simulink model "SF043A_TqOscn"  (R2013b)
settings: Solver=FixedStepDiscrete  SolverMode=SingleTasking  StartTime=0.0  StopTime=1  FixedStep=0.002  RelTol=1e-3
values from neighbouring files (symbols this model uses):
  ARCHGLBPRM_2MILLISEC_SEC_F32 = DataDict.Constant    [SF043A_TqOscn_DataDict.m]
  ARCHGLBPRM_2PI_ULS_F32 = DataDict.Constant    [SF043A_TqOscn_DataDict.m]
  DCTHD_MOTNWTMTR_F32 = DataDict.Constant    [SF043A_TqOscn_DataDict.m]
  DFTFALLRAMPRATE_MOTNWTMTRPERSEC_F32 = DataDict.Constant    [SF043A_TqOscn_DataDict.m]
  DFTPHAAGINC_MATRAD_F32 = DataDict.Constant    [SF043A_TqOscn_DataDict.m]
  DFTRISNGRAMPRATE_MOTNWTMTRPERSEC_F32 = DataDict.Constant    [SF043A_TqOscn_DataDict.m]
  FltInj_f32 = DataDict.Client    [SF043A_TqOscn_DataDict.m]
  FLTINJ_TQOSCN_PREFINALCMD = DataDict.Constant    [SF043A_TqOscn_DataDict.m]
  MAXAMP_MOTNWTMTR_F32 = DataDict.Constant    [SF043A_TqOscn_DataDict.m]
  MAXRAMPRATE_MOTNWTMTR_F32 = DataDict.Constant    [SF043A_TqOscn_DataDict.m]
  MINAMP_MOTNWTMTR_F32 = DataDict.Constant    [SF043A_TqOscn_DataDict.m]
  MINRAMPRATE_MOTNWTMTR_F32 = DataDict.Constant    [SF043A_TqOscn_DataDict.m]
  TqOscnAmpLimY = DataDict.Calibration    [SF043A_TqOscn_DataDict.m]
  TqOscnFallRampRateCal = DataDict.Calibration    [SF043A_TqOscn_DataDict.m]
  TqOscnFrqIn = DataDict.Calibration    [SF043A_TqOscn_DataDict.m]
  TqOscnRisngRampRateCal = DataDict.Calibration    [SF043A_TqOscn_DataDict.m]
  TqOscnUseRampRateCal = DataDict.Calibration    [SF043A_TqOscn_DataDict.m]
libraries: NxtrLim x6, simulink x3, NxtrAbslt x3, Fil x2, FixdToFloat x2, autosarlib x1, NxtrMath x1, FloatToFixd x1
(part 1 of 2)
settings Model: PauseTimes=0.5  Creator=hz69by  LastModifiedBy=HZ69BY
settings SolverCC: AutoInsertRateTranBlk=on  InsertRTBMode=Always
settings DataIOCC: LimitDataPoints=off  SaveFormat=Structure  ReturnWorkspaceOutputs=on
settings OptimizationCC: BlockReduction=off  InlineParams=on  ZeroExternalMemoryAtStartup=off  ZeroInternalMemoryAtStartup=off  OptimizeModelRefInitCode=on  LifeSpan=1
settings DebuggingCC: SignalInfNanChecking=error  SignalRangeChecking=warning  UnderspecifiedInitializationDetection=Simplified  SolverPrmCheckMsg=error  InheritedTsInSrcMsg=error  DiscreteInheritContinuousMsg=error  SingleTaskRateTransMsg=error  TasksWithSamePriorityMsg=error  SigSpecEnsureSampleTimeMsg=error  CheckMatrixSingularityMsg=error  ParameterUnderflowMsg=error  ParameterPrecisionLossMsg=error  ParameterTunabilityLossMsg=error  FixptConstUnderflowMsg=warning  FixptConstOverflowMsg=warning  VectorMatrixConversionMsg=error  SignalLabelMismatchMsg=error  UnconnectedInputMsg=error  UnconnectedOutputMsg=error  UnconnectedLineMsg=error  SFcnCompatibilityMsg=error  UniqueDataStoreMsg=warning  BusObjectLabelMismatch=error  RootOutportRequireBusObject=error  AssertControl=DisableAll  ModelReferenceIOMsg=error  ModelReferenceVersionMismatchMessage=warning  ModelReferenceIOMismatchMessage=error  ModelReferenceCSMismatchMessage=warning  ModelReferenceDataLoggingMessage=error  StateNameClashWarn=warning  StrictBusMsg=ErrorOnBusTreatedAsVector  NonBusSignalsTreatedAsBus=error  SFUnexpectedBacktrackingDiag=error  SFInvalidInputDataAccessInChartInitDiag=error  SFNoUnconditionalDefaultTransitionDiag=error  SFTransitionOutsideNaturalParentDiag=error  SFUnconditionalTransitionShadowingDiag=error  SFUndirectedBroadcastEventsDiag=error
settings ModelReferenceCC: ModelReferenceNumInstancesAllowed=Single
settings RTWCC: SystemTargetFile=autosar.tlc  GenCodeOnly=on  TemplateMakefile=ert_default_tmf  Description=AUTOSAR  GenerateReport=on  ProcessScript=autosar_make_rtw_hook  LaunchReport=on
settings CodeAppCC: GenerateComments=off  IgnoreCustomStorageClasses=off  CustomSymbolStrType=$N$R$M  CustomSymbolStrBlkIO=$N$M  SimulinkBlockComments=off
settings STFCustomTargetCC: ParMdlRefBuildCompliant=on  CompOptLevelCompliant=on  IncludeMdlTerminateFcn=off  CombineOutputUpdateFcns=on  SuppressErrorStatus=on  ERTFirstTimeCompliant=on  ERTCustomFileBanners=on  SupportNonFinite=off  SupportComplex=off  SupportContinuousTime=off  SupportNonInlinedSFcns=off  MATLABClassNameForMDSCustomization=Simulink.SoftwareTarget.ERTCustomization  AutosarCompliant=on  GRTInterface=off  SystemTargetFile=autosar.tlc
settings ERTTargetCC: CodeReplacementLibrary=ANSI_C  ConcurrentExecutionCompliant=off  IncludeMdlTerminateFcn=off  SuppressErrorStatus=on  SupportNonFinite=off  SupportComplex=off  ModelStepFunctionPrototypeControlCompliant=off  CPPClassGenCompliant=off  AutosarCompliant=on  InlinedParameterPlacement=NonHierarchical  ERTCustomFileTemplate=example_file_process.tlc  EnableUserReplacementTypes=on

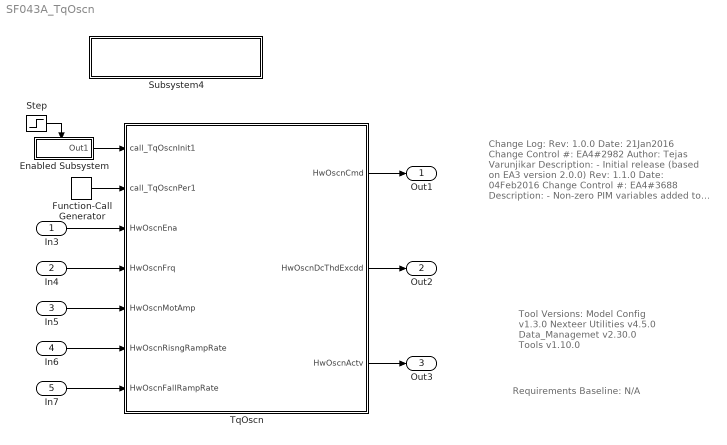
== system SF043A_TqOscn ==
  note: Change Log:
      |
      | Rev: 1.0.0
      | Date: 21Jan2016
      | Change Control #: EA4#2982
      | Author: Tejas Varunjikar
      | Description:
      | - Initial release (based on EA3 version 2.0.0)
      |
      | Rev: 1.1.0
      | Date: 04Feb2016
      | Change Control #: EA4#3688
      | Description:
      | - Non-zero PIM variables added to init
      | - Else logic updated inside "Angle Wrapper" subsystem
  note: Requirements Baseline: N/A
  note: Tool Versions:
      |
      | Model Config v1.3.0
      | Nexteer Utilities v4.5.0
      | Data_Managemet v2.30.0
      | Tools v1.10.0
  In3 : Inport  OutDataTypeStr=single
  In4 : Inport  Port=2  OutDataTypeStr=single
  In5 : Inport  Port=3  OutDataTypeStr=single
  In6 : Inport  Port=4  OutDataTypeStr=single
  In7 : Inport  Port=5  OutDataTypeStr=single
  Enabled Subsystem : Subsystem  TreatAsAtomicUnit=on
  Function-Call Generator : simulink/Ports & Subsystems/Function-Call Generator  sample_time=0.002  numberOfIterations=1
      settings: AttributesFormatString=%<sample_time>
  Step : Step  Time=0.002  Before=1  After=0  SampleTime=0
  Subsystem4 : Subsystem  Description=|  mask(Copyright Information){none=on}
      | Copyright info block.                                               
      |                                                                     
      | Place copyright information at the top of every subsystem in design.
      mask prompts: none "No parameters"
      mask help: Place copyright information at the top of every subsystem in design.
      mask Display:
      | NxtrConf = 'Nexteer Confidential';
      | 
      | sys = bdroot; %handle for the current model ("system")
      | first = get_param(sys,'Created');
      | first = first(end-3:end);  %year is last four digits
      | 
      | last = get_param(sys,'LastModifiedDate');
      | if isempty(last)
      |     last = datestr(now,'yyyy');
      | else
      |     last = last(end-3:end);
      | end
      | 
      | if strcmp(first,last)
      |     fprintf('%s\nCopyright  %s Nexteer',NxtrConf,first);
      | else
      |     fprintf('%s\n%s%s-%s Nexteer',NxtrConf,char(169),first,last);
      | end
  TqOscn : Subsystem
  Out1 : Outport
  Out2 : Outport  Port=2
  Out3 : Outport  Port=3
  wires:
  TqOscn/1(HwOscnCmd) -> Out1/1
  TqOscn/2(HwOscnDcThdExcdd) -> Out2/1
  TqOscn/3(HwOscnActv) -> Out3/1
  Enabled Subsystem/1(Out1) -> TqOscn/1(call_TqOscnInit1)
  Function-Call Generator/1 -> TqOscn/2(call_TqOscnPer1)
  Step/1 -> Enabled Subsystem/Enable
  In6/1 -> TqOscn/6(HwOscnRisngRampRate)
  In4/1 -> TqOscn/4(HwOscnFrq)
  In5/1 -> TqOscn/5(HwOscnMotAmp)
  In3/1 -> TqOscn/3(HwOscnEna)
  In7/1 -> TqOscn/7(HwOscnFallRampRate)

== system SF043A_TqOscn/Enabled Subsystem ==
  Enable : EnablePort
  Function-Call Generator : simulink/Ports & Subsystems/Function-Call Generator  sample_time=0.002  numberOfIterations=1
      settings: AttributesFormatString=%<sample_time>
  Out1 : Outport
  wires:
  Function-Call Generator/1 -> Out1/1

== system SF043A_TqOscn/Subsystem4 ==

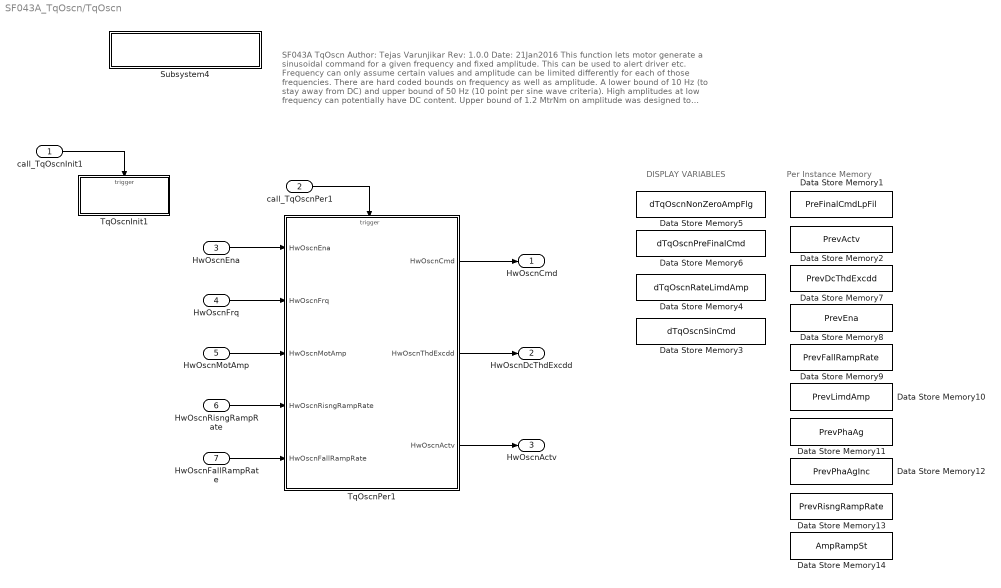
== system SF043A_TqOscn/TqOscn ==
  note: DISPLAY VARIABLES
  note: SF043A  TqOscn
      | Author: Tejas Varunjikar
      |
      | Rev: 1.0.0
      | Date: 21Jan2016
      |
      | This function lets motor generate a sinusoidal command for a given frequency and fixed amplitude.
      | This can be used to alert driver etc. Frequency can only assume certain values and amplitude can
      | be limited differently for each of those frequencies.
      | There are hard coded bounds on frequency as well as amplitude. A lower bound  of 10 Hz (to stay
      | away from DC) and upper bound of 50 Hz (10 point per sine wave criteria). High amplitudes at low
      | frequency can potentially have DC content. Upper bound of 1.2 MtrNm on amplitude was designed
      | to avoid more than ~3 HwNm DC content, and lower bound is just zero.
      | A simple DC Check block is included intended to turn off this function if DC signal exceeds ~3 HwNm.
  note: Per Instance Memory
  call_TqOscnInit1 : Inport
  call_TqOscnPer1 : Inport  Port=2
  HwOscnEna : Inport  Port=3
  HwOscnFrq : Inport  Port=4
  HwOscnMotAmp : Inport  Port=5
  HwOscnRisngRampRate : Inport  Port=6
  HwOscnFallRampRate : Inport  Port=7
  Data Store Memory1 : DataStoreMemory  DataStoreName=PreFinalCmdLpFil  InitialValue=[]  StateMustResolveToSignalObject=on
  Data Store Memory10 : DataStoreMemory  DataStoreName=PrevLimdAmp  WriteAfterWriteMsg=warning  StateMustResolveToSignalObject=on
  Data Store Memory11 : DataStoreMemory  DataStoreName=PrevPhaAg  WriteAfterWriteMsg=warning  StateMustResolveToSignalObject=on
  Data Store Memory12 : DataStoreMemory  DataStoreName=PrevPhaAgInc  WriteAfterWriteMsg=warning  StateMustResolveToSignalObject=on
  Data Store Memory13 : DataStoreMemory  DataStoreName=PrevRisngRampRate  WriteAfterWriteMsg=warning  StateMustResolveToSignalObject=on
  Data Store Memory14 : DataStoreMemory  DataStoreName=AmpRampSt  WriteAfterWriteMsg=warning  StateMustResolveToSignalObject=on
  Data Store Memory2 : DataStoreMemory  DataStoreName=PrevActv  WriteAfterWriteMsg=warning  StateMustResolveToSignalObject=on
  Data Store Memory3 : DataStoreMemory  DataStoreName=dTqOscnSinCmd  ReadBeforeWriteMsg=warning  WriteAfterWriteMsg=error  WriteAfterReadMsg=error  StateMustResolveToSignalObject=on
  Data Store Memory4 : DataStoreMemory  DataStoreName=dTqOscnRateLimdAmp  ReadBeforeWriteMsg=warning  WriteAfterWriteMsg=error  WriteAfterReadMsg=error  StateMustResolveToSignalObject=on
  Data Store Memory5 : DataStoreMemory  DataStoreName=dTqOscnNonZeroAmpFlg  ReadBeforeWriteMsg=warning  WriteAfterWriteMsg=error  WriteAfterReadMsg=error  StateMustResolveToSignalObject=on
  Data Store Memory6 : DataStoreMemory  DataStoreName=dTqOscnPreFinalCmd  ReadBeforeWriteMsg=warning  WriteAfterWriteMsg=error  WriteAfterReadMsg=error  StateMustResolveToSignalObject=on
  Data Store Memory7 : DataStoreMemory  DataStoreName=PrevDcThdExcdd  WriteAfterWriteMsg=warning  StateMustResolveToSignalObject=on
  Data Store Memory8 : DataStoreMemory  DataStoreName=PrevEna  WriteAfterWriteMsg=warning  StateMustResolveToSignalObject=on
  Data Store Memory9 : DataStoreMemory  DataStoreName=PrevFallRampRate  WriteAfterWriteMsg=warning  StateMustResolveToSignalObject=on
  Subsystem4 : Subsystem  Description=|  mask(Copyright Information){none=on}
      | Copyright info block.                                               
      |                                                                     
      | Place copyright information at the top of every subsystem in design.
      mask prompts: none "No parameters"
      mask help: Place copyright information at the top of every subsystem in design.
      mask Display:
      | NxtrConf = 'Nexteer Confidential';
      | 
      | sys = bdroot; %handle for the current model ("system")
      | first = get_param(sys,'Created');
      | first = first(end-3:end);  %year is last four digits
      | 
      | last = get_param(sys,'LastModifiedDate');
      | if isempty(last)
      |     last = datestr(now,'yyyy');
      | else
      |     last = last(end-3:end);
      | end
      | 
      | if strcmp(first,last)
      |     fprintf('%s\nCopyright  %s Nexteer',NxtrConf,first);
      | else
      |     fprintf('%s\n%s%s-%s Nexteer',NxtrConf,char(169),first,last);
      | end
  TqOscnInit1 : Subsystem  TreatAsAtomicUnit=on
  TqOscnPer1 : Subsystem  TreatAsAtomicUnit=on
  HwOscnCmd : Outport
  HwOscnDcThdExcdd : Outport  Port=2
  HwOscnActv : Outport  Port=3
  wires:
  HwOscnEna/1 -> TqOscnPer1/1(HwOscnEna)
  HwOscnFrq/1 -> TqOscnPer1/2(HwOscnFrq)
  HwOscnMotAmp/1 -> TqOscnPer1/3(HwOscnMotAmp)
  TqOscnPer1/1(HwOscnCmd) -> HwOscnCmd/1
  TqOscnPer1/2(HwOscnThdExcdd) -> HwOscnDcThdExcdd/1
  HwOscnFallRampRate/1 -> TqOscnPer1/5(HwOscnFallRampRate)
  HwOscnRisngRampRate/1 -> TqOscnPer1/4(HwOscnRisngRampRate)
  TqOscnPer1/3(HwOscnActv) -> HwOscnActv/1
  call_TqOscnPer1/1 -> TqOscnPer1/Trigger
  call_TqOscnInit1/1 -> TqOscnInit1/Trigger

== system SF043A_TqOscn/TqOscn/Subsystem4 ==

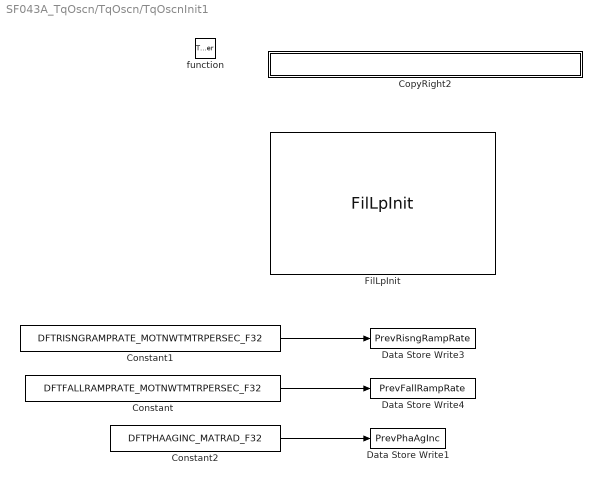
== system SF043A_TqOscn/TqOscn/TqOscnInit1 ==
  function : TriggerPort  TriggerType=function-call
  Constant : Constant  Value=DFTFALLRAMPRATE_MOTNWTMTRPERSEC_F32  OutDataTypeStr=single
  Constant1 : Constant  Value=DFTRISNGRAMPRATE_MOTNWTMTRPERSEC_F32  OutDataTypeStr=single
  Constant2 : Constant  Value=DFTPHAAGINC_MATRAD_F32  OutDataTypeStr=single
  CopyRight2 : Subsystem  Description=|  mask(Copyright Information){none=on}
      | Copyright info block.                                               
      |                                                                     
      | Place copyright information at the top of every subsystem in design.
      mask prompts: none "No parameters"
      mask help: Place copyright information at the top of every subsystem in design.
      mask Display:
      | NxtrConf = 'Nexteer Confidential';
      | 
      | sys = bdroot; %handle for the current model ("system")
      | first = get_param(sys,'Created');
      | if(isempty(first))
      |     first = datestr(now,'yyyy');
      | else
      |     first = first(end-3:end);  %year is last four digits
      | end
      | 
      | last = get_param(sys,'LastModifiedDate');
      | if isempty(last)
      |     last = datestr(now,'yyyy');
      | else
      |     last = last(end-3:end);
      | end
      | 
      | if strcmp(first,last)
      |     fprintf('%s -- Copyright %s Nexteer',NxtrConf,first)
      | else
      |     fprintf('%s -- %s%s- %s Nexteer',NxtrConf,char(169),first,last)
      | end
  Data Store Write1 : DataStoreWrite  DataStoreName=PrevPhaAgInc
  Data Store Write3 : DataStoreWrite  DataStoreName=PrevRisngRampRate
  Data Store Write4 : DataStoreWrite  DataStoreName=PrevFallRampRate
  FilLpInit : Fil/FilLpInit  Ic=0  Ts=ARCHGLBPRM_2MILLISEC_SEC_F32  Freq=DCCALCNLPFILFRQ_HZ_F32  StVar=PreFinalCmdLpFil
  wires:
  Constant/1 -> Data Store Write4/1
  Constant1/1 -> Data Store Write3/1
  Constant2/1 -> Data Store Write1/1

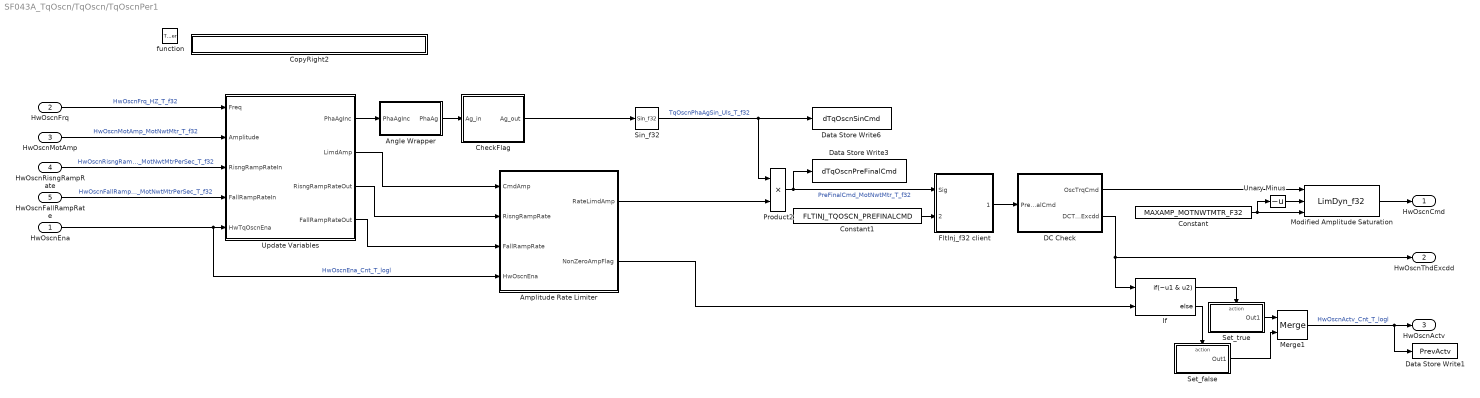
== system SF043A_TqOscn/TqOscn/TqOscnPer1 ==
  HwOscnEna : Inport
  HwOscnFrq : Inport  Port=2
  HwOscnMotAmp : Inport  Port=3
  HwOscnRisngRampRate : Inport  Port=4
  HwOscnFallRampRate : Inport  Port=5
  function : TriggerPort  TriggerType=function-call
  Amplitude Rate Limiter : Subsystem
  Angle Wrapper : Subsystem
  CheckFlag : Subsystem
  Constant : Constant  Value=MAXAMP_MOTNWTMTR_F32
  Constant1 : Constant  Value=FLTINJ_TQOSCN_PREFINALCMD
  CopyRight2 : Subsystem  Description=|  mask(Copyright Information){none=on}
      | Copyright info block.                                               
      |                                                                     
      | Place copyright information at the top of every subsystem in design.
      mask prompts: none "No parameters"
      mask help: Place copyright information at the top of every subsystem in design.
      mask Display:
      | NxtrConf = 'Nexteer Confidential';
      | 
      | sys = bdroot; %handle for the current model ("system")
      | first = get_param(sys,'Created');
      | if(isempty(first))
      |     first = datestr(now,'yyyy');
      | else
      |     first = first(end-3:end);  %year is last four digits
      | end
      | 
      | last = get_param(sys,'LastModifiedDate');
      | if isempty(last)
      |     last = datestr(now,'yyyy');
      | else
      |     last = last(end-3:end);
      | end
      | 
      | if strcmp(first,last)
      |     fprintf('%s -- Copyright %s Nexteer',NxtrConf,first)
      | else
      |     fprintf('%s -- %s%s- %s Nexteer',NxtrConf,char(169),first,last)
      | end
  DC Check : Subsystem
  Data Store Write1 : DataStoreWrite  DataStoreName=PrevActv
  Data Store Write3 : DataStoreWrite  DataStoreName=dTqOscnPreFinalCmd
  Data Store Write6 : DataStoreWrite  DataStoreName=dTqOscnSinCmd
  FltInj_f32 client : Subsystem  Variant=on
      settings: GeneratePreprocessorConditionals=on
  If : If  NumInputs=2  IfExpression=~u1 & u2
  Merge1 : Merge
  Modified Amplitude Saturation : NxtrLim/LimDyn_f32
  Product2 : Product  RndMeth=Zero
  Set_false : Subsystem  TreatAsAtomicUnit=on
  Set_true : Subsystem  TreatAsAtomicUnit=on
  Sin_f32 : NxtrMath/Sin_f32  SFunctionSpec=single y1 = Sin_f32(single u1)
      settings: AttributesFormatString=%<MaskType>
  Unary Minus : UnaryMinus
  Update Variables : Subsystem  TreatAsAtomicUnit=on
  HwOscnCmd : Outport
  HwOscnThdExcdd : Outport  Port=2
  HwOscnActv : Outport  Port=3
  wires:
  Constant/1 -> Modified Amplitude Saturation/3, Unary Minus/1
  Update Variables/2(LimdAmp) -> Amplitude Rate Limiter/1(CmdAmp)
  Modified Amplitude Saturation/1 -> HwOscnCmd/1
  Update Variables/1(PhaAgInc) -> Angle Wrapper/1(PhaAgInc)
  Unary Minus/1 -> Modified Amplitude Saturation/2
  Angle Wrapper/1(PhaAg) -> CheckFlag/1(Ag_in)
  Sin_f32/1 -> Product2/1, Data Store Write6/1  "TqOscnPhaAgSin_Uls_T_f32"
  CheckFlag/1(Ag_out) -> Sin_f32/1
  DC Check/1(OscTrqCmd) -> Modified Amplitude Saturation/1
  DC Check/2(DCThdExcdd) -> HwOscnThdExcdd/1, If/1
  HwOscnFrq/1 -> Update Variables/1(Freq)  "HwOscnFrq_HZ_T_f32"
  Amplitude Rate Limiter/1(RateLimdAmp) -> Product2/2
  Amplitude Rate Limiter/2(NonZeroAmpFlag) -> If/2
  Merge1/1 -> HwOscnActv/1, Data Store Write1/1  "HwOscnActv_Cnt_T_logl"
  HwOscnRisngRampRate/1 -> Update Variables/3(RisngRampRateIn)  "HwOscnRisngRampRate_MotNwtMtrPerSec_T_f32"
  HwOscnFallRampRate/1 -> Update Variables/4(FallRampRateIn)  "HwOscnFallRampRate_MotNwtMtrPerSec_T_f32"
  HwOscnMotAmp/1 -> Update Variables/2(Amplitude)  "HwOscnMotAmp_MotNwtMtr_T_f32"
  Update Variables/3(RisngRampRateOut) -> Amplitude Rate Limiter/2(RisngRampRate)
  Update Variables/4(FallRampRateOut) -> Amplitude Rate Limiter/3(FallRampRate)
  FltInj_f32 client/1(Sig_Out) -> DC Check/1(PreFinalCmd)
  Product2/1 -> Data Store Write3/1, FltInj_f32 client/1(Sig)  "PreFinalCmd_MotNwtMtr_T_f32"
  Constant1/1 -> FltInj_f32 client/2("LocnKey  ")
  HwOscnEna/1 -> Amplitude Rate Limiter/4(HwOscnEna), Update Variables/5(HwTqOscnEna)  "HwOscnEna_Cnt_T_logl"
  If/1 -> Set_true/Action
  If/2 -> Set_false/Action
  Set_true/1(Out1) -> Merge1/1
  Set_false/1(Out1) -> Merge1/2

== system SF043A_TqOscn/TqOscn/TqOscnInit1/CopyRight2 ==

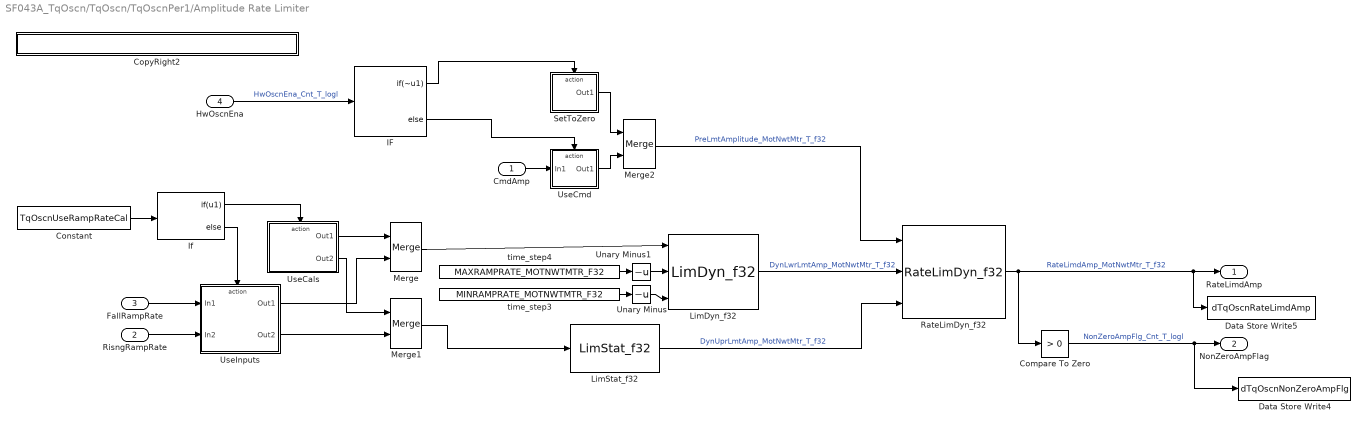
== system SF043A_TqOscn/TqOscn/TqOscnPer1/Amplitude Rate Limiter ==
  CmdAmp : Inport
  RisngRampRate : Inport  Port=2
  FallRampRate : Inport  Port=3
  HwOscnEna : Inport  Port=4
  Compare To Zero : simulink/Logic and Bit Operations/Compare To Zero  relop=>  OutDataTypeStr=boolean
  Constant : Constant  Value=TqOscnUseRampRateCal
  CopyRight2 : Subsystem  Description=|  mask(Copyright Information){none=on}
      | Copyright info block.                                               
      |                                                                     
      | Place copyright information at the top of every subsystem in design.
      mask prompts: none "No parameters"
      mask help: Place copyright information at the top of every subsystem in design.
      mask Display:
      | NxtrConf = 'Nexteer Confidential';
      | 
      | sys = bdroot; %handle for the current model ("system")
      | first = get_param(sys,'Created');
      | if(isempty(first))
      |     first = datestr(now,'yyyy');
      | else
      |     first = first(end-3:end);  %year is last four digits
      | end
      | 
      | last = get_param(sys,'LastModifiedDate');
      | if isempty(last)
      |     last = datestr(now,'yyyy');
      | else
      |     last = last(end-3:end);
      | end
      | 
      | if strcmp(first,last)
      |     fprintf('%s -- Copyright %s Nexteer',NxtrConf,first)
      | else
      |     fprintf('%s -- %s%s- %s Nexteer',NxtrConf,char(169),first,last)
      | end
  Data Store Write4 : DataStoreWrite  DataStoreName=dTqOscnNonZeroAmpFlg
  Data Store Write5 : DataStoreWrite  DataStoreName=dTqOscnRateLimdAmp
  IF : If  IfExpression=~u1
  If : If  IfExpression=u1
  LimDyn_f32 : NxtrLim/LimDyn_f32
  LimStat_f32 : NxtrLim/LimStat_f32  LoLim=MINRAMPRATE_MOTNWTMTR_F32  HiLim=MAXRAMPRATE_MOTNWTMTR_F32
      settings: AttributesFormatString=|
      | Low Limit: %<LoLim>
      | High Limit:%<HiLim>
  Merge : Merge
  Merge1 : Merge
  Merge2 : Merge
  RateLimDyn_f32 : NxtrLim/RateLimDyn_f32  StVar=AmpRampSt  Ts=ARCHGLBPRM_2MILLISEC_SEC_F32
      settings: AttributesFormatString=StVar: %<StVar>
  SetToZero : Subsystem  TreatAsAtomicUnit=on
  Unary Minus : UnaryMinus
  Unary Minus1 : UnaryMinus
  UseCals : Subsystem  TreatAsAtomicUnit=on
  UseCmd : Subsystem  TreatAsAtomicUnit=on
  UseInputs : Subsystem  TreatAsAtomicUnit=on
  time_step3 : Constant  Value=MINRAMPRATE_MOTNWTMTR_F32
  time_step4 : Constant  Value=MAXRAMPRATE_MOTNWTMTR_F32
  RateLimdAmp : Outport
  NonZeroAmpFlag : Outport  Port=2
  wires:
  RateLimDyn_f32/1 -> Data Store Write5/1, RateLimdAmp/1, Compare To Zero/1  "RateLimdAmp_MotNwtMtr_T_f32"
  Constant/1 -> If/1
  If/2 -> UseInputs/Action
  If/1 -> UseCals/Action
  FallRampRate/1 -> UseInputs/1(In1)
  RisngRampRate/1 -> UseInputs/2(In2)
  UseInputs/1(Out1) -> Merge/2
  UseCals/1(Out1) -> Merge/1
  UseCals/2(Out2) -> Merge1/1
  UseInputs/2(Out2) -> Merge1/2
  Merge2/1 -> RateLimDyn_f32/1  "PreLmtAmplitude_MotNwtMtr_T_f32"
  Compare To Zero/1 -> NonZeroAmpFlag/1, Data Store Write4/1  "NonZeroAmpFlg_Cnt_T_logl"
  Merge1/1 -> LimStat_f32/1
  LimStat_f32/1 -> RateLimDyn_f32/3  "DynUprLmtAmp_MotNwtMtr_T_f32"
  Merge/1 -> LimDyn_f32/1
  LimDyn_f32/1 -> RateLimDyn_f32/2  "DynLwrLmtAmp_MotNwtMtr_T_f32"
  time_step4/1 -> Unary Minus1/1
  time_step3/1 -> Unary Minus/1
  HwOscnEna/1 -> IF/1  "HwOscnEna_Cnt_T_logl"
  IF/1 -> SetToZero/Action
  IF/2 -> UseCmd/Action
  SetToZero/1(Out1) -> Merge2/1
  UseCmd/1(Out1) -> Merge2/2
  CmdAmp/1 -> UseCmd/1(In1)
  Unary Minus1/1 -> LimDyn_f32/2
  Unary Minus/1 -> LimDyn_f32/3

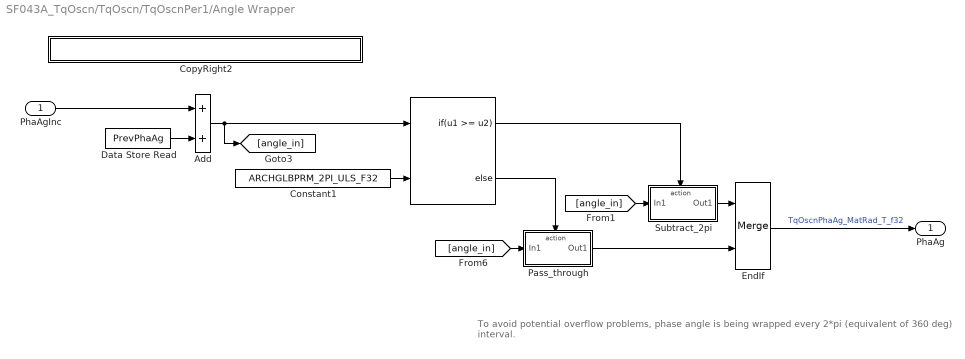
== system SF043A_TqOscn/TqOscn/TqOscnPer1/Angle Wrapper ==
  note: To avoid potential overflow problems, phase angle is being wrapped every 2*pi (equivalent of 360 deg) interval.
  PhaAgInc : Inport
  " " : If  NumInputs=2  IfExpression=u1 >= u2
  Add : Sum
  Constant1 : Constant  Value=ARCHGLBPRM_2PI_ULS_F32
  CopyRight2 : Subsystem  Description=|  mask(Copyright Information){none=on}
      | Copyright info block.                                               
      |                                                                     
      | Place copyright information at the top of every subsystem in design.
      mask prompts: none "No parameters"
      mask help: Place copyright information at the top of every subsystem in design.
      mask Display:
      | NxtrConf = 'Nexteer Confidential';
      | 
      | sys = bdroot; %handle for the current model ("system")
      | first = get_param(sys,'Created');
      | if(isempty(first))
      |     first = datestr(now,'yyyy');
      | else
      |     first = first(end-3:end);  %year is last four digits
      | end
      | 
      | last = get_param(sys,'LastModifiedDate');
      | if isempty(last)
      |     last = datestr(now,'yyyy');
      | else
      |     last = last(end-3:end);
      | end
      | 
      | if strcmp(first,last)
      |     fprintf('%s -- Copyright %s Nexteer',NxtrConf,first)
      | else
      |     fprintf('%s -- %s%s- %s Nexteer',NxtrConf,char(169),first,last)
      | end
  Data Store Read : DataStoreRead  DataStoreName=PrevPhaAg
  EndIf : Merge
  Pass_through : Subsystem  TreatAsAtomicUnit=on
  Subtract_2pi : Subsystem  TreatAsAtomicUnit=on
  PhaAg : Outport
  wires:
  " "/1 -> Subtract_2pi/Action
  Subtract_2pi/1(Out1) -> EndIf/1
  Pass_through/1(Out1) -> EndIf/2
  [angle_in] -> Pass_through/1(In1)
  " "/2 -> Pass_through/Action
  PhaAgInc/1 -> Add/1
  [angle_in] -> Subtract_2pi/1(In1)
  EndIf/1 -> PhaAg/1  "TqOscnPhaAg_MatRad_T_f32"
  Constant1/1 -> " "/2
  Add/1 -> [angle_in], " "/1
  Data Store Read/1 -> Add/2

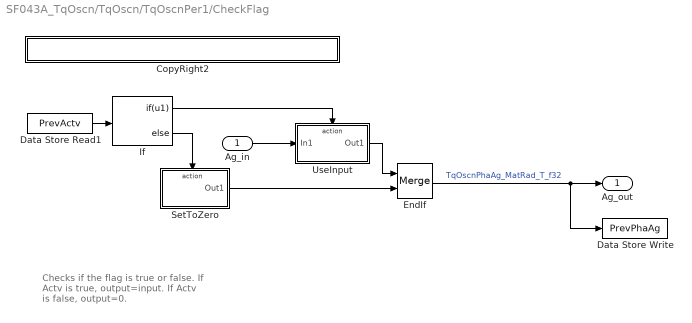
== system SF043A_TqOscn/TqOscn/TqOscnPer1/CheckFlag ==
  note: Checks if the flag is true or false.
      | If Actv is true,  output=input.
      | If Actv is false, output=0.
  Ag_in : Inport
  CopyRight2 : Subsystem  Description=|  mask(Copyright Information){none=on}
      | Copyright info block.                                               
      |                                                                     
      | Place copyright information at the top of every subsystem in design.
      mask prompts: none "No parameters"
      mask help: Place copyright information at the top of every subsystem in design.
      mask Display:
      | NxtrConf = 'Nexteer Confidential';
      | 
      | sys = bdroot; %handle for the current model ("system")
      | first = get_param(sys,'Created');
      | if(isempty(first))
      |     first = datestr(now,'yyyy');
      | else
      |     first = first(end-3:end);  %year is last four digits
      | end
      | 
      | last = get_param(sys,'LastModifiedDate');
      | if isempty(last)
      |     last = datestr(now,'yyyy');
      | else
      |     last = last(end-3:end);
      | end
      | 
      | if strcmp(first,last)
      |     fprintf('%s -- Copyright %s Nexteer',NxtrConf,first)
      | else
      |     fprintf('%s -- %s%s- %s Nexteer',NxtrConf,char(169),first,last)
      | end
  Data Store Read1 : DataStoreRead  DataStoreName=PrevActv
  Data Store Write : DataStoreWrite  DataStoreName=PrevPhaAg
  EndIf : Merge
  If : If  IfExpression=u1
  SetToZero : Subsystem  TreatAsAtomicUnit=on
  UseInput : Subsystem  TreatAsAtomicUnit=on
  Ag_out : Outport
  wires:
  If/1 -> UseInput/Action
  UseInput/1(Out1) -> EndIf/1
  SetToZero/1(Out1) -> EndIf/2
  If/2 -> SetToZero/Action
  Data Store Read1/1 -> If/1
  EndIf/1 -> Data Store Write/1, Ag_out/1  "TqOscnPhaAg_MatRad_T_f32"
  Ag_in/1 -> UseInput/1(In1)

== system SF043A_TqOscn/TqOscn/TqOscnPer1/CopyRight2 ==

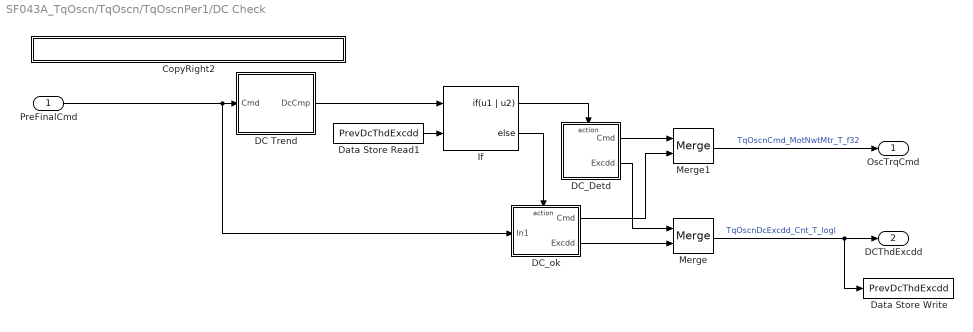
== system SF043A_TqOscn/TqOscn/TqOscnPer1/DC Check ==
  PreFinalCmd : Inport
  CopyRight2 : Subsystem  Description=|  mask(Copyright Information){none=on}
      | Copyright info block.                                               
      |                                                                     
      | Place copyright information at the top of every subsystem in design.
      mask prompts: none "No parameters"
      mask help: Place copyright information at the top of every subsystem in design.
      mask Display:
      | NxtrConf = 'Nexteer Confidential';
      | 
      | sys = bdroot; %handle for the current model ("system")
      | first = get_param(sys,'Created');
      | if(isempty(first))
      |     first = datestr(now,'yyyy');
      | else
      |     first = first(end-3:end);  %year is last four digits
      | end
      | 
      | last = get_param(sys,'LastModifiedDate');
      | if isempty(last)
      |     last = datestr(now,'yyyy');
      | else
      |     last = last(end-3:end);
      | end
      | 
      | if strcmp(first,last)
      |     fprintf('%s -- Copyright %s Nexteer',NxtrConf,first)
      | else
      |     fprintf('%s -- %s%s- %s Nexteer',NxtrConf,char(169),first,last)
      | end
  DC Trend : Subsystem
  DC_Detd : Subsystem  TreatAsAtomicUnit=on
  DC_ok : Subsystem  TreatAsAtomicUnit=on
  Data Store Read1 : DataStoreRead  DataStoreName=PrevDcThdExcdd
  Data Store Write : DataStoreWrite  DataStoreName=PrevDcThdExcdd
  If : If  NumInputs=2  IfExpression=u1 | u2
  Merge : Merge
  Merge1 : Merge
  OscTrqCmd : Outport
  DCThdExcdd : Outport  Port=2
  wires:
  PreFinalCmd/1 -> DC_ok/1(In1), DC Trend/1(Cmd)
  Data Store Read1/1 -> If/2
  DC Trend/1(DcCmp) -> If/1
  If/1 -> DC_Detd/Action
  Merge/1 -> Data Store Write/1, DCThdExcdd/1  "TqOscnDcExcdd_Cnt_T_logl"
  Merge1/1 -> OscTrqCmd/1  "TqOscnCmd_MotNwtMtr_T_f32"
  DC_Detd/1(Cmd) -> Merge1/1
  DC_ok/1(Cmd) -> Merge1/2
  DC_Detd/2(Excdd) -> Merge/1
  DC_ok/2(Excdd) -> Merge/2
  If/2 -> DC_ok/Action

== system SF043A_TqOscn/TqOscn/TqOscnPer1/FltInj_f32 client ==
  note: Created Aug 18, 2015
      | Kevin Derry
  note: 1) Only subsystems can be added as variant choices at this level
      | 2) Blocks cannot be connected at this level as connectivity is
      | automatically determined at simulation, based on the active variant
  note: FltInj_f32
  Sig : Inport  OutDataTypeStr=single
  "LocnKey  " : Inport  Port=2  OutDataTypeStr=uint16
  CodeGen : Subsystem  VariantControl=FLTINJENA == STD_ON
  CopyRight1 : Subsystem  Description=|  mask(Copyright Information){none=on}
      | Copyright info block.                                               
      |                                                                     
      | Place copyright information at the top of every subsystem in design.
      mask prompts: none "No parameters"
      mask help: Place copyright information at the top of every subsystem in design.
      mask Display:
      | NxtrConf = 'Nexteer Confidential';
      | 
      | sys = bdroot; %handle for the current model ("system")
      | first = get_param(sys,'Created');
      | if(isempty(first))
      |     first = datestr(now,'yyyy');
      | else
      |     first = first(end-3:end);  %year is last four digits
      | end
      | 
      | last = get_param(sys,'LastModifiedDate');
      | if isempty(last)
      |     last = datestr(now,'yyyy');
      | else
      |     last = last(end-3:end);
      | end
      | 
      | if strcmp(first,last)
      |     fprintf('%s -- Copyright %s Nexteer',NxtrConf,first)
      | else
      |     fprintf('%s -- %s%s- %s Nexteer',NxtrConf,char(169),first,last)
      | end
  Sim : Subsystem  TreatAsAtomicUnit=on  VariantControl=FLTINJENA ~= STD_ON  mask(Fault_Injection){}
      mask help: Simulation mode is just a pass-thru.
  Sig_Out : Outport  OutDataTypeStr=single

== system SF043A_TqOscn/TqOscn/TqOscnPer1/Set_false ==
  Action Port : ActionPort  ActionType=else
  Constant : Constant  Value=false  OutDataTypeStr=boolean
      settings: AttributesFormatString=%<OutDataTypeStr>
  CopyRight2 : Subsystem  Description=|  mask(Copyright Information){none=on}
      | Copyright info block.                                               
      |                                                                     
      | Place copyright information at the top of every subsystem in design.
      mask prompts: none "No parameters"
      mask help: Place copyright information at the top of every subsystem in design.
      mask Display:
      | NxtrConf = 'Nexteer Confidential';
      | 
      | sys = bdroot; %handle for the current model ("system")
      | first = get_param(sys,'Created');
      | if(isempty(first))
      |     first = datestr(now,'yyyy');
      | else
      |     first = first(end-3:end);  %year is last four digits
      | end
      | 
      | last = get_param(sys,'LastModifiedDate');
      | if isempty(last)
      |     last = datestr(now,'yyyy');
      | else
      |     last = last(end-3:end);
      | end
      | 
      | if strcmp(first,last)
      |     fprintf('%s -- Copyright %s Nexteer',NxtrConf,first)
      | else
      |     fprintf('%s -- %s%s- %s Nexteer',NxtrConf,char(169),first,last)
      | end
  Out1 : Outport
  wires:
  Constant/1 -> Out1/1

== system SF043A_TqOscn/TqOscn/TqOscnPer1/Set_true ==
  Action Port : ActionPort  ActionType=then
  Constant : Constant  Value=true  OutDataTypeStr=boolean
      settings: AttributesFormatString=%<OutDataTypeStr>
  CopyRight2 : Subsystem  Description=|  mask(Copyright Information){none=on}
      | Copyright info block.                                               
      |                                                                     
      | Place copyright information at the top of every subsystem in design.
      mask prompts: none "No parameters"
      mask help: Place copyright information at the top of every subsystem in design.
      mask Display:
      | NxtrConf = 'Nexteer Confidential';
      | 
      | sys = bdroot; %handle for the current model ("system")
      | first = get_param(sys,'Created');
      | if(isempty(first))
      |     first = datestr(now,'yyyy');
      | else
      |     first = first(end-3:end);  %year is last four digits
      | end
      | 
      | last = get_param(sys,'LastModifiedDate');
      | if isempty(last)
      |     last = datestr(now,'yyyy');
      | else
      |     last = last(end-3:end);
      | end
      | 
      | if strcmp(first,last)
      |     fprintf('%s -- Copyright %s Nexteer',NxtrConf,first)
      | else
      |     fprintf('%s -- %s%s- %s Nexteer',NxtrConf,char(169),first,last)
      | end
  Out1 : Outport
  wires:
  Constant/1 -> Out1/1

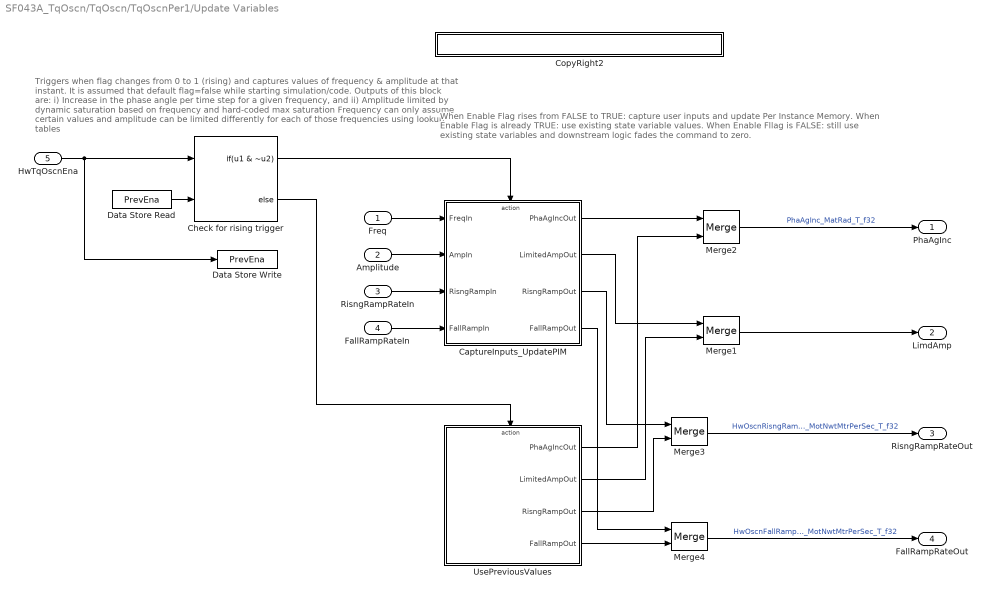
== system SF043A_TqOscn/TqOscn/TqOscnPer1/Update Variables ==
  note: Triggers when flag changes from 0 to 1 (rising) and captures values of frequency & amplitude at
      |  that instant. It is assumed that default flag=false while starting simulation/code.
      | Outputs of this block are: i) Increase in the phase angle per time step for a given frequency, and
      | ii) Amplitude limited by dynamic saturation based on frequency and hard-coded max saturation
      |
      | Frequency can only assume certain values and amplitude can be limited differently for each of
      |  those frequencies using lookup tables
  note: When Enable Flag rises from FALSE to TRUE:  capture user inputs and update Per Instance Memory.
      | When Enable Flag is already TRUE:  use existing state variable values.
      | When Enable Fllag is FALSE:  still use existing state variables and downstream logic fades the command to zero.
  Freq : Inport
  Amplitude : Inport  Port=2
  RisngRampRateIn : Inport  Port=3
  FallRampRateIn : Inport  Port=4
  HwTqOscnEna : Inport  Port=5
  CaptureInputs_UpdatePIM : Subsystem
  Check for rising trigger : If  NumInputs=2  IfExpression=u1 & ~u2
  CopyRight2 : Subsystem  Description=|  mask(Copyright Information){none=on}
      | Copyright info block.                                               
      |                                                                     
      | Place copyright information at the top of every subsystem in design.
      mask prompts: none "No parameters"
      mask help: Place copyright information at the top of every subsystem in design.
      mask Display:
      | NxtrConf = 'Nexteer Confidential';
      | 
      | sys = bdroot; %handle for the current model ("system")
      | first = get_param(sys,'Created');
      | if(isempty(first))
      |     first = datestr(now,'yyyy');
      | else
      |     first = first(end-3:end);  %year is last four digits
      | end
      | 
      | last = get_param(sys,'LastModifiedDate');
      | if isempty(last)
      |     last = datestr(now,'yyyy');
      | else
      |     last = last(end-3:end);
      | end
      | 
      | if strcmp(first,last)
      |     fprintf('%s -- Copyright %s Nexteer',NxtrConf,first)
      | else
      |     fprintf('%s -- %s%s- %s Nexteer',NxtrConf,char(169),first,last)
      | end
  Data Store Read : DataStoreRead  Priority=1  DataStoreName=PrevEna
      settings: AttributesFormatString=priority: %<Priority>
  Data Store Write : DataStoreWrite  Priority=2  DataStoreName=PrevEna
      settings: AttributesFormatString=priority: %<Priority>
  Merge{1..4} (4 alike) : Merge
  UsePreviousValues : Subsystem
  PhaAgInc : Outport
  LimdAmp : Outport  Port=2
  RisngRampRateOut : Outport  Port=3
  FallRampRateOut : Outport  Port=4
  wires:
  HwTqOscnEna/1 -> Data Store Write/1, Check for rising trigger/1
  Check for rising trigger/1 -> CaptureInputs_UpdatePIM/Action
  Check for rising trigger/2 -> UsePreviousValues/Action
  Data Store Read/1 -> Check for rising trigger/2
  Freq/1 -> CaptureInputs_UpdatePIM/1(FreqIn)
  Amplitude/1 -> CaptureInputs_UpdatePIM/2(AmpIn)
  FallRampRateIn/1 -> CaptureInputs_UpdatePIM/4(FallRampIn)
  RisngRampRateIn/1 -> CaptureInputs_UpdatePIM/3(RisngRampIn)
  CaptureInputs_UpdatePIM/1(PhaAgIncOut) -> Merge2/1
  CaptureInputs_UpdatePIM/2(LimitedAmpOut) -> Merge1/1
  CaptureInputs_UpdatePIM/3(RisngRampOut) -> Merge3/1
  CaptureInputs_UpdatePIM/4(FallRampOut) -> Merge4/1
  UsePreviousValues/1(PhaAgIncOut) -> Merge2/2
  UsePreviousValues/2(LimitedAmpOut) -> Merge1/2
  UsePreviousValues/3(RisngRampOut) -> Merge3/2
  UsePreviousValues/4(FallRampOut) -> Merge4/2
  Merge2/1 -> PhaAgInc/1  "PhaAgInc_MatRad_T_f32"
  Merge1/1 -> LimdAmp/1
  Merge3/1 -> RisngRampRateOut/1  "HwOscnRisngRampRate_MotNwtMtrPerSec_T_f32"
  Merge4/1 -> FallRampRateOut/1  "HwOscnFallRampRate_MotNwtMtrPerSec_T_f32"

== system SF043A_TqOscn/TqOscn/TqOscnPer1/Amplitude Rate Limiter/CopyRight2 ==

== system SF043A_TqOscn/TqOscn/TqOscnPer1/Amplitude Rate Limiter/SetToZero ==
  Action Port : ActionPort  ActionType=then
  Constant4 : Constant  Value=0  OutDataTypeStr=single
      settings: AttributesFormatString=%<OutDataTypeStr>
  CopyRight2 : Subsystem  Description=|  mask(Copyright Information){none=on}
      | Copyright info block.                                               
      |                                                                     
      | Place copyright information at the top of every subsystem in design.
      mask prompts: none "No parameters"
      mask help: Place copyright information at the top of every subsystem in design.
      mask Display:
      | NxtrConf = 'Nexteer Confidential';
      | 
      | sys = bdroot; %handle for the current model ("system")
      | first = get_param(sys,'Created');
      | if(isempty(first))
      |     first = datestr(now,'yyyy');
      | else
      |     first = first(end-3:end);  %year is last four digits
      | end
      | 
      | last = get_param(sys,'LastModifiedDate');
      | if isempty(last)
      |     last = datestr(now,'yyyy');
      | else
      |     last = last(end-3:end);
      | end
      | 
      | if strcmp(first,last)
      |     fprintf('%s -- Copyright %s Nexteer',NxtrConf,first)
      | else
      |     fprintf('%s -- %s%s- %s Nexteer',NxtrConf,char(169),first,last)
      | end
  Out1 : Outport
  wires:
  Constant4/1 -> Out1/1

== system SF043A_TqOscn/TqOscn/TqOscnPer1/Amplitude Rate Limiter/UseCals ==
  Action Port : ActionPort  ActionType=then
  Constant1 : Constant  Value=TqOscnRisngRampRateCal
  Constant2 : Constant  Value=TqOscnFallRampRateCal
  CopyRight2 : Subsystem  Description=|  mask(Copyright Information){none=on}
      | Copyright info block.                                               
      |                                                                     
      | Place copyright information at the top of every subsystem in design.
      mask prompts: none "No parameters"
      mask help: Place copyright information at the top of every subsystem in design.
      mask Display:
      | NxtrConf = 'Nexteer Confidential';
      | 
      | sys = bdroot; %handle for the current model ("system")
      | first = get_param(sys,'Created');
      | if(isempty(first))
      |     first = datestr(now,'yyyy');
      | else
      |     first = first(end-3:end);  %year is last four digits
      | end
      | 
      | last = get_param(sys,'LastModifiedDate');
      | if isempty(last)
      |     last = datestr(now,'yyyy');
      | else
      |     last = last(end-3:end);
      | end
      | 
      | if strcmp(first,last)
      |     fprintf('%s -- Copyright %s Nexteer',NxtrConf,first)
      | else
      |     fprintf('%s -- %s%s- %s Nexteer',NxtrConf,char(169),first,last)
      | end
  Out1 : Outport
  Out2 : Outport  Port=2
  wires:
  Constant2/1 -> Out1/1
  Constant1/1 -> Out2/1

== system SF043A_TqOscn/TqOscn/TqOscnPer1/Amplitude Rate Limiter/UseCmd ==
  In1 : Inport
  Action Port : ActionPort  ActionType=else
  Out1 : Outport
  wires:
  In1/1 -> Out1/1

== system SF043A_TqOscn/TqOscn/TqOscnPer1/Amplitude Rate Limiter/UseInputs ==
  In1 : Inport
  In2 : Inport  Port=2
  Action Port : ActionPort  ActionType=else
  Out1 : Outport
  Out2 : Outport  Port=2
  wires:
  In2/1 -> Out2/1
  In1/1 -> Out1/1

== system SF043A_TqOscn/TqOscn/TqOscnPer1/Angle Wrapper/CopyRight2 ==

== system SF043A_TqOscn/TqOscn/TqOscnPer1/Angle Wrapper/Pass_through ==
  In1 : Inport
  Action Port : ActionPort  ActionType=else
  CopyRight2 : Subsystem  Description=|  mask(Copyright Information){none=on}
      | Copyright info block.                                               
      |                                                                     
      | Place copyright information at the top of every subsystem in design.
      mask prompts: none "No parameters"
      mask help: Place copyright information at the top of every subsystem in design.
      mask Display:
      | NxtrConf = 'Nexteer Confidential';
      | 
      | sys = bdroot; %handle for the current model ("system")
      | first = get_param(sys,'Created');
      | if(isempty(first))
      |     first = datestr(now,'yyyy');
      | else
      |     first = first(end-3:end);  %year is last four digits
      | end
      | 
      | last = get_param(sys,'LastModifiedDate');
      | if isempty(last)
      |     last = datestr(now,'yyyy');
      | else
      |     last = last(end-3:end);
      | end
      | 
      | if strcmp(first,last)
      |     fprintf('%s -- Copyright %s Nexteer',NxtrConf,first)
      | else
      |     fprintf('%s -- %s%s- %s Nexteer',NxtrConf,char(169),first,last)
      | end
  Out1 : Outport
  wires:
  In1/1 -> Out1/1

== system SF043A_TqOscn/TqOscn/TqOscnPer1/Angle Wrapper/Subtract_2pi ==
  In1 : Inport
  Action Port : ActionPort  ActionType=then
  Constant : Constant  Value=ARCHGLBPRM_2PI_ULS_F32
  CopyRight2 : Subsystem  Description=|  mask(Copyright Information){none=on}
      | Copyright info block.                                               
      |                                                                     
      | Place copyright information at the top of every subsystem in design.
      mask prompts: none "No parameters"
      mask help: Place copyright information at the top of every subsystem in design.
      mask Display:
      | NxtrConf = 'Nexteer Confidential';
      | 
      | sys = bdroot; %handle for the current model ("system")
      | first = get_param(sys,'Created');
      | if(isempty(first))
      |     first = datestr(now,'yyyy');
      | else
      |     first = first(end-3:end);  %year is last four digits
      | end
      | 
      | last = get_param(sys,'LastModifiedDate');
      | if isempty(last)
      |     last = datestr(now,'yyyy');
      | else
      |     last = last(end-3:end);
      | end
      | 
      | if strcmp(first,last)
      |     fprintf('%s -- Copyright %s Nexteer',NxtrConf,first)
      | else
      |     fprintf('%s -- %s%s- %s Nexteer',NxtrConf,char(169),first,last)
      | end
  Subtract : Sum  Inputs=+-
  Out1 : Outport
  wires:
  In1/1 -> Subtract/1
  Subtract/1 -> Out1/1
  Constant/1 -> Subtract/2

== system SF043A_TqOscn/TqOscn/TqOscnPer1/CheckFlag/CopyRight2 ==

== system SF043A_TqOscn/TqOscn/TqOscnPer1/CheckFlag/SetToZero ==
  Action Port : ActionPort  ActionType=else
  Constant2 : Constant  Value=0  OutDataTypeStr=single
      settings: AttributesFormatString=%<OutDataTypeStr>
  CopyRight2 : Subsystem  Description=|  mask(Copyright Information){none=on}
      | Copyright info block.                                               
      |                                                                     
      | Place copyright information at the top of every subsystem in design.
      mask prompts: none "No parameters"
      mask help: Place copyright information at the top of every subsystem in design.
      mask Display:
      | NxtrConf = 'Nexteer Confidential';
      | 
      | sys = bdroot; %handle for the current model ("system")
      | first = get_param(sys,'Created');
      | if(isempty(first))
      |     first = datestr(now,'yyyy');
      | else
      |     first = first(end-3:end);  %year is last four digits
      | end
      | 
      | last = get_param(sys,'LastModifiedDate');
      | if isempty(last)
      |     last = datestr(now,'yyyy');
      | else
      |     last = last(end-3:end);
      | end
      | 
      | if strcmp(first,last)
      |     fprintf('%s -- Copyright %s Nexteer',NxtrConf,first)
      | else
      |     fprintf('%s -- %s%s- %s Nexteer',NxtrConf,char(169),first,last)
      | end
  Out1 : Outport
  wires:
  Constant2/1 -> Out1/1

== system SF043A_TqOscn/TqOscn/TqOscnPer1/CheckFlag/UseInput ==
  In1 : Inport
  Action Port : ActionPort  ActionType=then
  CopyRight2 : Subsystem  Description=|  mask(Copyright Information){none=on}
      | Copyright info block.                                               
      |                                                                     
      | Place copyright information at the top of every subsystem in design.
      mask prompts: none "No parameters"
      mask help: Place copyright information at the top of every subsystem in design.
      mask Display:
      | NxtrConf = 'Nexteer Confidential';
      | 
      | sys = bdroot; %handle for the current model ("system")
      | first = get_param(sys,'Created');
      | if(isempty(first))
      |     first = datestr(now,'yyyy');
      | else
      |     first = first(end-3:end);  %year is last four digits
      | end
      | 
      | last = get_param(sys,'LastModifiedDate');
      | if isempty(last)
      |     last = datestr(now,'yyyy');
      | else
      |     last = last(end-3:end);
      | end
      | 
      | if strcmp(first,last)
      |     fprintf('%s -- Copyright %s Nexteer',NxtrConf,first)
      | else
      |     fprintf('%s -- %s%s- %s Nexteer',NxtrConf,char(169),first,last)
      | end
  Out1 : Outport
  wires:
  In1/1 -> Out1/1

== system SF043A_TqOscn/TqOscn/TqOscnPer1/DC Check/CopyRight2 ==

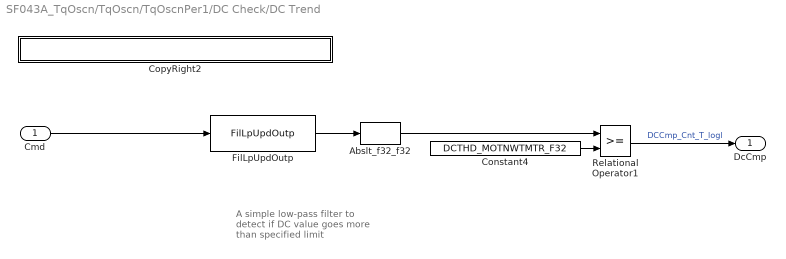
== system SF043A_TqOscn/TqOscn/TqOscnPer1/DC Check/DC Trend ==
  note: A simple low-pass filter to detect if DC value goes more than specified limit
  Cmd : Inport
  Abslt_f32_f32 : NxtrAbslt/Abslt_f32_f32  SFunctionSpec=single y1 = Abslt_f32_f32(single u1)
      settings: AttributesFormatString=%<Name>
  Constant4 : Constant  Value=DCTHD_MOTNWTMTR_F32
  CopyRight2 : Subsystem  Description=|  mask(Copyright Information){none=on}
      | Copyright info block.                                               
      |                                                                     
      | Place copyright information at the top of every subsystem in design.
      mask prompts: none "No parameters"
      mask help: Place copyright information at the top of every subsystem in design.
      mask Display:
      | NxtrConf = 'Nexteer Confidential';
      | 
      | sys = bdroot; %handle for the current model ("system")
      | first = get_param(sys,'Created');
      | if(isempty(first))
      |     first = datestr(now,'yyyy');
      | else
      |     first = first(end-3:end);  %year is last four digits
      | end
      | 
      | last = get_param(sys,'LastModifiedDate');
      | if isempty(last)
      |     last = datestr(now,'yyyy');
      | else
      |     last = last(end-3:end);
      | end
      | 
      | if strcmp(first,last)
      |     fprintf('%s -- Copyright %s Nexteer',NxtrConf,first)
      | else
      |     fprintf('%s -- %s%s- %s Nexteer',NxtrConf,char(169),first,last)
      | end
  FilLpUpdOutp : Fil/FilLpUpdOutp  StVar=PreFinalCmdLpFil
      settings: AttributesFormatString=StVar: %<StVar>
  Relational Operator1 : RelationalOperator  OutDataTypeStr=boolean
  DcCmp : Outport
  wires:
  FilLpUpdOutp/1 -> Abslt_f32_f32/1
  Constant4/1 -> Relational Operator1/2
  Relational Operator1/1 -> DcCmp/1  "DCCmp_Cnt_T_logl"
  Abslt_f32_f32/1 -> Relational Operator1/1
  Cmd/1 -> FilLpUpdOutp/1

== system SF043A_TqOscn/TqOscn/TqOscnPer1/DC Check/DC_Detd ==
  Action Port : ActionPort  ActionType=then
  Constant : Constant  Value=0  OutDataTypeStr=single
      settings: AttributesFormatString=%<OutDataTypeStr>
  Constant1 : Constant  Value=true  OutDataTypeStr=boolean
      settings: AttributesFormatString=%<OutDataTypeStr>
  CopyRight2 : Subsystem  Description=|  mask(Copyright Information){none=on}
      | Copyright info block.                                               
      |                                                                     
      | Place copyright information at the top of every subsystem in design.
      mask prompts: none "No parameters"
      mask help: Place copyright information at the top of every subsystem in design.
      mask Display:
      | NxtrConf = 'Nexteer Confidential';
      | 
      | sys = bdroot; %handle for the current model ("system")
      | first = get_param(sys,'Created');
      | if(isempty(first))
      |     first = datestr(now,'yyyy');
      | else
      |     first = first(end-3:end);  %year is last four digits
      | end
      | 
      | last = get_param(sys,'LastModifiedDate');
      | if isempty(last)
      |     last = datestr(now,'yyyy');
      | else
      |     last = last(end-3:end);
      | end
      | 
      | if strcmp(first,last)
      |     fprintf('%s -- Copyright %s Nexteer',NxtrConf,first)
      | else
      |     fprintf('%s -- %s%s- %s Nexteer',NxtrConf,char(169),first,last)
      | end
  Cmd : Outport
  Excdd : Outport  Port=2
  wires:
  Constant/1 -> Cmd/1
  Constant1/1 -> Excdd/1
